simulink model "hw11_1"  (R2018a)
settings: Solver=FixedStepAuto  StartTime=0.0  StopTime=5  FixedStep=.1  RelTol=1e-3
settings Model: Creator=mean_booty  LastModifiedBy=mean_booty

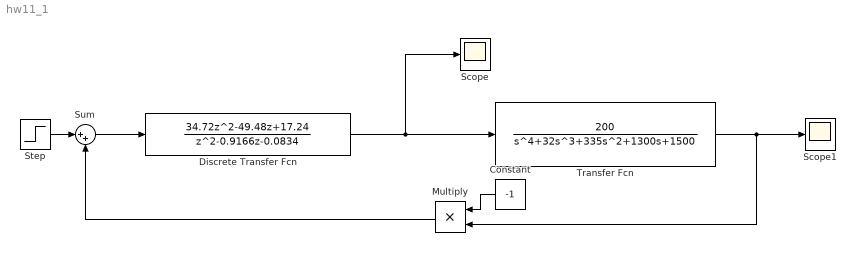
== system hw11_1 ==
  Constant : Constant  Value=-1
  Discrete Transfer Fcn : DiscreteTransferFcn  Numerator=[34.72 -49.48 17.24]  Denominator=[1 -0.9166 -0.0834]
  Multiply : Product
  Scope : Scope
  Scope1 : Scope
  Step : Step  Time=0  SampleTime=0
  Sum : Sum  Inputs=|++
  Transfer Fcn : TransferFcn  Numerator=[200]  Denominator=[1 32 335 1300 1500]
  wires:
  Step/1 -> Sum/1
  Multiply/1 -> Sum/2
  Constant/1 -> Multiply/1
  Sum/1 -> Discrete Transfer Fcn/1
  Discrete Transfer Fcn/1 -> Transfer Fcn/1, Scope/1
  Transfer Fcn/1 -> Multiply/2, Scope1/1
